simulink model "multi__micro1primarysecondarynn2"  (R2015a)
settings: Solver=ode23tb  StartTime=0.0  StopTime=2
model workspace: external: MAT-File D:\google drive\project\nn1\matla.mat (data not in the file)
undefined symbols (not defined in the file): cf, gam, gamp, k1, k2, k3, k5, Lc, lf, mp1, Mu, nq1, rc, sig, sigp, td, wn
libraries: powerlib x116, powerlib_meascontrol x32, powerlib_extras x2
(part 2 of 3)

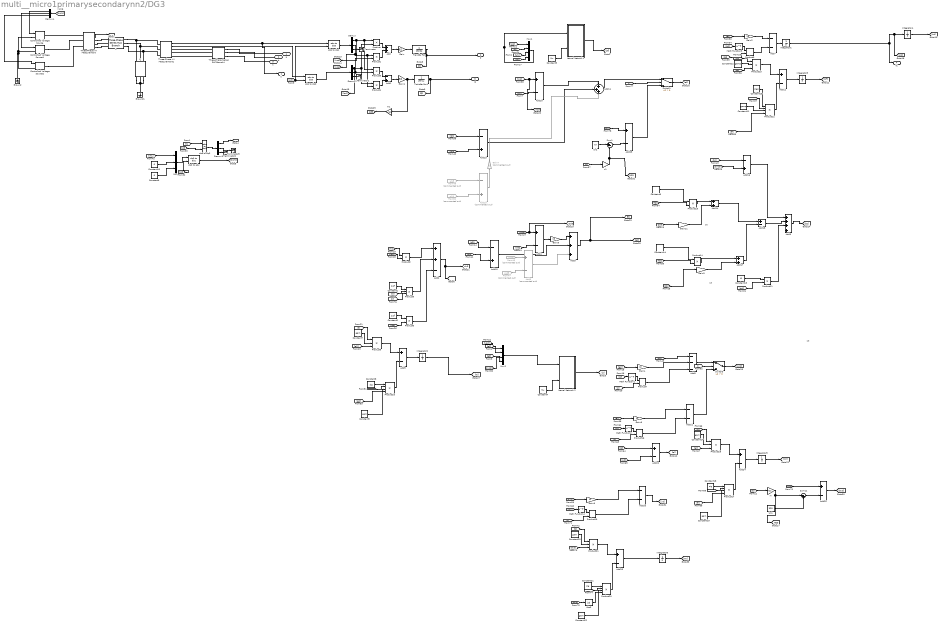
== system multi__micro1primarysecondarynn2/DG3 ==
  note: SE
  note: SE
  note: SE
  Abs3 : Abs
  Add : Sum
  Add{1,13,15..16} (4 alike) : Sum  Inputs=-+
  Add{4,9..10,12,18,22..26} (10 alike) : Sum  Inputs=+-
  Add11 : Sum  Inputs=+++
  Add14 : Sum
  Add17 : Sum
  Add19 : Sum  Commented=on  Inputs=-+
  Add2 : Sum  Inputs=++-
  Add20 : Sum  Inputs=--
  Add21 : Sum  Inputs=--
  Add3 : Sum  Inputs=+++
  Add5 : Sum  Inputs=++++
  Add6 : Sum  Commented=on  Inputs=+-
  Add7 : Sum  Inputs=--
  Add8 : Sum  Inputs=---
  C : powerlib/Elements/Three-Phase Series RLC Branch  LConnTagsString=A|B|C  RConnTagsString=A|B|C  BranchType=C  Resistance=1  Inductance=1e-3  Capacitance=cf  Measurements=None
  Constant1 : Constant  Value=1/cf
  Constant10 : Constant  Value=0
  Constant11 : Constant  Value=gamp
  Constant12 : Constant  Value=gamp
  Constant13 : Constant  Value=sigp
  Constant14 : Constant  Value=-31.446
  Constant15 : Constant  Value=k1
  Constant{7,9,17,19..20,22} (6 alike) : Constant  Value=gam
  Constant18 : Constant  Value=sig
  Constant2 : Constant  Value=1/cf
  Constant21 : Constant  Value=sig
  Constant3 : Constant  Value=Mu
  Constant4 : Constant  Value=Mu
  Constant5 : Constant  Value=-31.446
  Constant6 : Constant  Value=0
  Constant8 : Constant  Value=sig
  Controlled Voltage Source : powerlib/Electrical Sources/Controlled Voltage Source  Initialize=on  Source_Type=AC  Amplitude=0  Phase=0  Frequency=0  Measurements=None
  Controlled Voltage Source1 : powerlib/Electrical Sources/Controlled Voltage Source  Initialize=on  Source_Type=AC  Amplitude=0  Phase=0  Frequency=0  Measurements=None
  Controlled Voltage Source2 : powerlib/Electrical Sources/Controlled Voltage Source  Initialize=on  Source_Type=AC  Amplitude=0  Phase=0  Frequency=0  Measurements=None
  Demux{,1,3..4} (4 alike) : Demux  Outputs=3
  From46 : From  Commented=on  GotoTag=vod
  From47 : From  Commented=on  GotoTag=vod8
  From49 : From  Commented=on  GotoTag=w18  TagVisibility=global
  From52 : From  Commented=on  GotoTag=w11  TagVisibility=global
  Gain : Gain  Gain=3/2
  Gain1 : Gain  Gain=3/2
  Gain11 : Gain  Gain=31.446
  Gain2 : Gain  Gain=k3
  Gain3 : Gain  Gain=31.446
  Gain4 : Gain  Gain=k2
  Gain5 : Gain  Gain=k5
  Gain7 : Gain  Commented=on  Gain=k5
  Gain8 : Gain  Gain=k2
  Gain9 : Gain  Gain=k2
  Ground : powerlib/Elements/Ground  LConnTagsString=a
  Ground1 : powerlib/Elements/Ground  LConnTagsString=a
  Integrator1 : Integrator  UpperSaturationLimit=321  LowerSaturationLimit=314.16
  Integrator{2..3,5..6} (4 alike) : Integrator  InitialCondition=zeros(16,1)  UpperSaturationLimit=314.16  ZeroCross=off
  Integrator4 : Integrator  UpperSaturationLimit=314.16  ZeroCross=off
  L : powerlib/Elements/Three-Phase Series RLC Branch  LConnTagsString=A|B|C  RConnTagsString=A|B|C  BranchType=RL  Resistance=0.1  Inductance=lf  Capacitance=1e-6  Measurements=None
  Math Function{1..4} (4 alike) : Math  Operator=transpose  OutputSignalType=real  SaturateOnIntegerOverflow=on
  Mux : Mux  Inputs=3
  Mux1 : Mux
  Mux2 : Mux
  Neural Network 1 : MATLAB Function  TreatAsAtomicUnit=on
  Neural Network 2 : MATLAB Function  TreatAsAtomicUnit=on
  Product{,1,3..4} (4 alike) : Product  RndMeth=Zero
  Product{10,12,17,20} (4 alike) : Product  Inputs=4
  Product{2,6,11,14..15} (5 alike) : Product
  Product{5,8,13,18,21} (5 alike) : Product  Inputs=3
  Product{7,9,16,19} (4 alike) : Product  Multiplication=Matrix(*)
  Sum1 : Sum  Inputs=|+-
  Sum11 : Sum  Inputs=|-+
  Switch1 : Switch  Criteria=u2 > Threshold
  Switch3 : Switch  Criteria=u2 > Threshold
  Terminator{,1..3} (4 alike) : Terminator
  Three-Phase Series RLC Branch4 : powerlib/Elements/Three-Phase Series RLC Branch  LConnTagsString=A|B|C  RConnTagsString=A|B|C  BranchType=RL  Resistance=rc  Inductance=Lc  Capacitance=1e-6  Measurements=None
  Three-Phase V-I Measurement : powerlib/Measurements/Three-Phase V-I Measurement  VoltageMeasurement=phase-to-ground  SetLabelV=off  LabelV=Vabc  Vpu=off  VpuLL=off  CurrentMeasurement=yes  SetLabelI=off  LabelI=Iabc  Ipu=off  Pbase=100e6  Vbase=500e3  OutputType=Complex  PhasorSimulation=off  PSBequivalent=0
  Three-Phase V-I Measurement1 : powerlib/Measurements/Three-Phase V-I Measurement  VoltageMeasurement=phase-to-ground  SetLabelV=off  LabelV=Vabc  Vpu=off  VpuLL=off  CurrentMeasurement=yes  SetLabelI=off  LabelI=Iabc  Ipu=off  Pbase=100e6  Vbase=500e3  OutputType=Complex  PhasorSimulation=off  PSBequivalent=0
  Transfer Fcn : TransferFcn  Denominator=[td 1]
  Transfer Fcn1 : TransferFcn  Denominator=[td 1]
  Un1 : Constant  Value=325
  Un2 : Constant  Value=wn
  abc to dq0 : powerlib_meascontrol/Transformations/abc to dq0  Alignment=90 degrees behind phase A axis
  abc to dq1 : powerlib_meascontrol/Transformations/abc to dq0  Alignment=90 degrees behind phase A axis
  abc to dq3 : powerlib_meascontrol/Transformations/abc to dq0  Alignment=90 degrees behind phase A axis
  dq0 to abc : powerlib_meascontrol/Transformations/dq0 to abc  Alignment=90 degrees behind phase A axis
  m : Gain  Gain=nq1
  m1 : Gain  Gain=nq1
  n1 : Gain  Gain=mp1
  a : PMIOPort  Tag=PMCPort  Port=1  Side=Right
  b : PMIOPort  Tag=PMCPort  Port=2  Side=Right
  c : PMIOPort  Tag=PMCPort  Port=3  Side=Right
  U : Outport
  P : Outport  Port=2
  Q : Outport  Port=3
  f1 : Outport  Port=4
  tag scope: E3=global, MP3=global, NQ3=global, Q33=global, dv3=global, vod3=global, w13=global
  wires:
  [PWM] -> Demux4/1
  Three-Phase V-I Measurement1/1 -> U/1, abc to dq1/1
  Demux/1 -> [vod], Product/1, Product3/1
  Demux1/1 -> [iod], Product/2, Product4/1
  Demux/2 -> [voq], Product1/1, Product4/2
  Demux1/2 -> Product1/2, Product3/2
  Product/1 -> Add/1
  Product1/1 -> Add/2
  Product3/1 -> Add1/1
  Product4/1 -> Add1/2
  [wt] -> abc to dq1/2, abc to dq0/2
  Demux4/1 -> Controlled Voltage Source/1
  Demux4/2 -> Controlled Voltage Source1/1
  Demux4/3 -> Controlled Voltage Source2/1
  Three-Phase V-I Measurement/2 -> [IL]
  Add/1 -> Gain/1
  Gain/1 -> Transfer Fcn/1
  Add1/1 -> Gain1/1
  Gain1/1 -> m1/1, Transfer Fcn1/1
  abc to dq1/1 -> Demux/1
  abc to dq0/1 -> Demux1/1
  Demux/3 -> Terminator/1
  Demux1/3 -> Terminator1/1
  [vod] -> [vod3], Add4/1
  Gain4/1 -> Add8/2
  [e2] -> Gain4/1
  [S] -> Product7/2
  [W] -> Math Function1/1
  Math Function1/1 -> Product7/1
  Product7/1 -> Add8/3
  [S] -> Product8/1
  Constant7/1 -> Product8/2
  [e2] -> Product8/3
  Product8/1 -> Add9/1
  Constant8/1 -> Product10/1
  [W] -> Product10/2
  Product10/1 -> Add9/2
  Constant9/1 -> Product10/3
  Add9/1 -> Integrator2/1
  [vod2] -> Add4/2
  [IL] -> abc to dq3/1
  Demux3/1 -> [Id]
  Demux3/2 -> Terminator3/1
  [wt] -> abc to dq3/2
  Mux/1 -> dq0 to abc/1
  [wt] -> dq0 to abc/2
  abc to dq3/1 -> Demux3/1
  dq0 to abc/1 -> [PWM]
  Demux3/3 -> Terminator2/1
  [vn1] -> Mux/1
  Constant10/1 -> Mux/2
  Constant6/1 -> Mux/3
  Transfer Fcn/1 -> P/1, [P]
  Transfer Fcn1/1 -> Q/1, [Q]
  [w1] -> Mux1/1
  [ef] -> Mux1/2
  [w1] -> Mux1/3
  [MP2] -> Mux1/4
  [w1] -> [w13], Add10/1
  [w12] -> Add10/2
  [Sf] -> Product13/1
  Constant12/1 -> Product13/2
  [ef] -> Product13/3
  Product13/1 -> Add12/1
  Constant13/1 -> Product12/1
  [Wf] -> Product12/2
  Product12/1 -> Add12/2
  Constant11/1 -> Product12/3
  Add12/1 -> Integrator3/1
  Integrator3/1 -> [Wf]
  Three-Phase V-I Measurement1/2 -> abc to dq0/1
  Add10/1 -> Add11/1
  [MP2] -> Add13/1
  [MP3] -> Add13/2
  Add13/1 -> Add11/2
  [NQ2] -> Add15/1
  [NQ3] -> Add15/2
  Add15/1 -> Add3/2
  [e1] -> Add8/1
  Add4/1 -> Gain5/1
  Gain5/1 -> Add3/1
  [vod] -> Mux2/1
  [e1] -> Mux2/2
  [dvodi] -> Mux2/3
  [e2] -> Mux2/4
  Constant5/1 -> Product15/1
  [NQ3] -> Product15/2
  Product15/1 -> Add14/1
  [Q33] -> Gain11/1
  Constant14/1 -> Product14/1
  [NQ2] -> Product14/2
  Product14/1 -> Add17/1
  [Q22] -> Gain3/1
  Add17/1 -> Add18/2
  Add14/1 -> Add18/1
  Gain3/1 -> Add17/2
  Gain11/1 -> Add14/2
  Add18/1 -> Add5/2
  Constant15/1 -> Product11/1
  [e1] -> Product11/2
  Product11/1 -> Add5/3
  [dv2] -> Add16/1
  Add16/1 -> Add5/1
  [dvodi] -> Add16/2
  From46/1 -> Add6/1
  From47/1 -> Add6/2
  Add6/1 -> Add3/3
  m1/1 -> [Q33]
  From49/1 -> Add19/1
  From52/1 -> Add19/2
  Add19/1 -> Gain7/1
  Gain7/1 -> Add11/3
  Neural Network 1/1(Sz1) -> [Sf]
  [e2] -> Product10/4
  [ef] -> Gain2/1
  [Sf] -> Product9/2
  [Wf] -> Math Function3/1
  Math Function3/1 -> Product9/1
  Gain2/1 -> Add7/1
  Product9/1 -> Add7/2
  Add7/1 -> Integrator1/1
  [ef] -> Product12/4
  Neural Network 2/1(Sz1) -> [S]
  Constant4/1 -> Neural Network 2/2(mu)
  Mux2/1 -> Neural Network 2/1(X)
  Constant3/1 -> Neural Network 1/2(mu)
  Mux1/1 -> Neural Network 1/1(X)
  Add3/1 -> [E3], [e1]
  Add5/1 -> [e2]
  Integrator4/1 -> [wt]
  [ti] -> Switch3/2
  Add8/1 -> Switch3/1
  Switch3/1 -> [vn1]
  [el] -> Gain8/1
  [S] -> Product16/2
  [Wl] -> Math Function2/1
  Math Function2/1 -> Product16/1
  Product16/1 -> Add21/2
  Gain8/1 -> Add21/1
  Add21/1 -> Switch3/3
  [Id] -> Add22/1
  [vd] -> Add22/2
  Add22/1 -> [el]
  [S] -> Product18/1
  Constant17/1 -> Product18/2
  [el] -> Product18/3
  Product18/1 -> Add24/1
  Constant18/1 -> Product17/1
  [Wl] -> Product17/2
  Product17/1 -> Add24/2
  Constant19/1 -> Product17/3
  Add24/1 -> Integrator5/1
  Integrator5/1 -> [Wl]
  [el] -> Product17/4
  [vod] -> Add25/1
  Add25/1 -> [evd]
  Sum11/1 -> Add25/2
  [Q] -> m/1
  Un1/1 -> Sum11/2
  m/1 -> [NQ3], Sum11/1
  [evd] -> Gain9/1
  [S] -> Product19/2
  [Wv] -> Math Function4/1
  Math Function4/1 -> Product19/1
  Product19/1 -> Add20/2
  Gain9/1 -> Add20/1
  Add20/1 -> [vd]
  [S] -> Product21/1
  Constant20/1 -> Product21/2
  [evd] -> Product21/3
  Product21/1 -> Add26/1
  Constant21/1 -> Product20/1
  [Wl] -> Product20/2
  Product20/1 -> Add26/2
  Constant22/1 -> Product20/3
  Abs3/1 -> Product20/4
  [evd] -> Abs3/1
  Add26/1 -> Integrator6/1
  Integrator6/1 -> [Wv]
  Integrator2/1 -> [W]
  [w1] -> Product2/1
  [voq] -> Product2/2
  Product2/1 -> Add2/1
  Constant1/1 -> Product5/1
  [Id] -> Product5/2
  Product5/1 -> Add2/2
  Constant2/1 -> Product6/1
  [iod] -> Product6/2
  Product6/1 -> Add2/3
  Add2/1 -> [dvodi], [dv3]
  [rr] -> Product5/3
  Integrator1/1 -> [w1], Integrator4/1, f1/1
  [P] -> n1/1
  Un2/1 -> Sum1/1  "f"
  n1/1 -> [MP3], Sum1/2
  Sum1/1 -> Add23/2
  [w1] -> Add23/1
  Add11/1 -> Switch1/1
  [ti] -> Switch1/2
  Switch1/1 -> [ef]
  Add23/1 -> Switch1/3
  connections:
  C/RConn1 -- Ground1/LConn1 -- C/RConn3 -- C/RConn2
  L/RConn2 -- Three-Phase V-I Measurement1/LConn2 -- C/LConn2
  L/RConn1 -- Three-Phase V-I Measurement1/LConn1 -- C/LConn1
  L/RConn3 -- Three-Phase V-I Measurement1/LConn3 -- C/LConn3
  Controlled Voltage Source/LConn1 -- Controlled Voltage Source1/LConn1 -- Ground/LConn1 -- Controlled Voltage Source2/LConn1
  Three-Phase V-I Measurement/LConn1 -- Controlled Voltage Source/RConn1
  Controlled Voltage Source1/RConn1 -- Three-Phase V-I Measurement/LConn2
  Controlled Voltage Source2/RConn1 -- Three-Phase V-I Measurement/LConn3
  Three-Phase V-I Measurement/RConn1 -- L/LConn1
  Three-Phase V-I Measurement/RConn2 -- L/LConn2
  Three-Phase V-I Measurement/RConn3 -- L/LConn3
  Three-Phase Series RLC Branch4/RConn1 -- Three-Phase V-I Measurement1/RConn1
  Three-Phase Series RLC Branch4/RConn2 -- Three-Phase V-I Measurement1/RConn2
  Three-Phase Series RLC Branch4/RConn3 -- Three-Phase V-I Measurement1/RConn3
  Three-Phase Series RLC Branch4/LConn3 -- c/RConn1
  Three-Phase Series RLC Branch4/LConn2 -- b/RConn1
  Three-Phase Series RLC Branch4/LConn1 -- a/RConn1

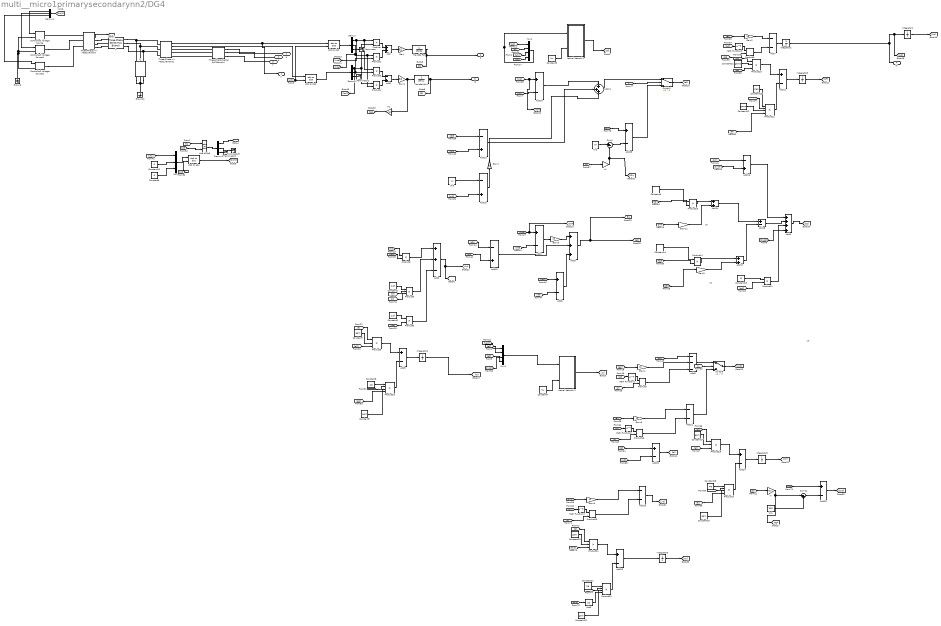
== system multi__micro1primarysecondarynn2/DG4 ==
  note: SE
  note: SE
  note: SE
  Abs3 : Abs
  Add : Sum
  Add{1,13,15..16,19} (5 alike) : Sum  Inputs=-+
  Add{4,6,9..10,12,18,22..26} (11 alike) : Sum  Inputs=+-
  Add11 : Sum  Inputs=+++
  Add14 : Sum
  Add17 : Sum
  Add2 : Sum  Inputs=++-
  Add20 : Sum  Inputs=--
  Add21 : Sum  Inputs=--
  Add3 : Sum  Inputs=+++
  Add5 : Sum  Inputs=++++
  Add7 : Sum  Inputs=--
  Add8 : Sum  Inputs=---
  C : powerlib/Elements/Three-Phase Series RLC Branch  LConnTagsString=A|B|C  RConnTagsString=A|B|C  BranchType=C  Resistance=1  Inductance=1e-3  Capacitance=cf  Measurements=None
  Constant1 : Constant  Value=1/cf
  Constant10 : Constant  Value=0
  Constant11 : Constant  Value=gamp
  Constant12 : Constant  Value=gamp
  Constant13 : Constant  Value=sigp
  Constant14 : Constant  Value=-31.446
  Constant15 : Constant  Value=k1
  Constant{7,9,17,19..20,22} (6 alike) : Constant  Value=gam
  Constant18 : Constant  Value=sig
  Constant2 : Constant  Value=1/cf
  Constant21 : Constant  Value=sig
  Constant3 : Constant  Value=Mu
  Constant4 : Constant  Value=Mu
  Constant5 : Constant  Value=-31.446
  Constant6 : Constant  Value=0
  Constant8 : Constant  Value=sig
  Controlled Voltage Source : powerlib/Electrical Sources/Controlled Voltage Source  Initialize=on  Source_Type=AC  Amplitude=0  Phase=0  Frequency=0  Measurements=None
  Controlled Voltage Source1 : powerlib/Electrical Sources/Controlled Voltage Source  Initialize=on  Source_Type=AC  Amplitude=0  Phase=0  Frequency=0  Measurements=None
  Controlled Voltage Source2 : powerlib/Electrical Sources/Controlled Voltage Source  Initialize=on  Source_Type=AC  Amplitude=0  Phase=0  Frequency=0  Measurements=None
  Demux{,1,3..4} (4 alike) : Demux  Outputs=3
  Gain : Gain  Gain=3/2
  Gain1 : Gain  Gain=3/2
  Gain11 : Gain  Gain=31.446
  Gain2 : Gain  Gain=k3
  Gain3 : Gain  Gain=31.446
  Gain4 : Gain  Gain=k2
  Gain5 : Gain  Gain=k5
  Gain7 : Gain  Gain=k5
  Gain8 : Gain  Gain=k2
  Gain9 : Gain  Gain=k2
  Ground : powerlib/Elements/Ground  LConnTagsString=a
  Ground1 : powerlib/Elements/Ground  LConnTagsString=a
  Integrator1 : Integrator  UpperSaturationLimit=321  LowerSaturationLimit=314.16
  Integrator{2..3,5..6} (4 alike) : Integrator  InitialCondition=zeros(16,1)  UpperSaturationLimit=314.16  ZeroCross=off
  Integrator4 : Integrator  UpperSaturationLimit=314.16  ZeroCross=off
  L : powerlib/Elements/Three-Phase Series RLC Branch  LConnTagsString=A|B|C  RConnTagsString=A|B|C  BranchType=RL  Resistance=0.1  Inductance=lf  Capacitance=1e-6  Measurements=None
  Math Function{1..4} (4 alike) : Math  Operator=transpose  OutputSignalType=real  SaturateOnIntegerOverflow=on
  Mux : Mux  Inputs=3
  Mux1 : Mux
  Mux2 : Mux
  Neural Network 1 : MATLAB Function  TreatAsAtomicUnit=on
  Neural Network 2 : MATLAB Function  TreatAsAtomicUnit=on
  Product{,1,3..4} (4 alike) : Product  RndMeth=Zero
  Product{10,12,17,20} (4 alike) : Product  Inputs=4
  Product{2,6,11,14..15} (5 alike) : Product
  Product{5,8,13,18,21} (5 alike) : Product  Inputs=3
  Product{7,9,16,19} (4 alike) : Product  Multiplication=Matrix(*)
  Sum1 : Sum  Inputs=|+-
  Sum11 : Sum  Inputs=|-+
  Switch1 : Switch  Criteria=u2 > Threshold
  Switch3 : Switch  Criteria=u2 > Threshold
  Terminator{,1..3} (4 alike) : Terminator
  Three-Phase Series RLC Branch4 : powerlib/Elements/Three-Phase Series RLC Branch  LConnTagsString=A|B|C  RConnTagsString=A|B|C  BranchType=RL  Resistance=rc  Inductance=Lc  Capacitance=1e-6  Measurements=None
  Three-Phase V-I Measurement : powerlib/Measurements/Three-Phase V-I Measurement  VoltageMeasurement=phase-to-ground  SetLabelV=off  LabelV=Vabc  Vpu=off  VpuLL=off  CurrentMeasurement=yes  SetLabelI=off  LabelI=Iabc  Ipu=off  Pbase=100e6  Vbase=500e3  OutputType=Complex  PhasorSimulation=off  PSBequivalent=0
  Three-Phase V-I Measurement1 : powerlib/Measurements/Three-Phase V-I Measurement  VoltageMeasurement=phase-to-ground  SetLabelV=off  LabelV=Vabc  Vpu=off  VpuLL=off  CurrentMeasurement=yes  SetLabelI=off  LabelI=Iabc  Ipu=off  Pbase=100e6  Vbase=500e3  OutputType=Complex  PhasorSimulation=off  PSBequivalent=0
  Transfer Fcn : TransferFcn  Denominator=[td 1]
  Transfer Fcn1 : TransferFcn  Denominator=[td 1]
  Un1 : Constant  Value=325
  Un2 : Constant  Value=wn
  Un3 : Constant  Value=wn
  abc to dq0 : powerlib_meascontrol/Transformations/abc to dq0  Alignment=90 degrees behind phase A axis
  abc to dq1 : powerlib_meascontrol/Transformations/abc to dq0  Alignment=90 degrees behind phase A axis
  abc to dq3 : powerlib_meascontrol/Transformations/abc to dq0  Alignment=90 degrees behind phase A axis
  dq0 to abc : powerlib_meascontrol/Transformations/dq0 to abc  Alignment=90 degrees behind phase A axis
  m : Gain  Gain=nq1
  m1 : Gain  Gain=nq1
  n1 : Gain  Gain=mp1
  a : PMIOPort  Tag=PMCPort  Port=1  Side=Right
  b : PMIOPort  Tag=PMCPort  Port=2  Side=Right
  c : PMIOPort  Tag=PMCPort  Port=3  Side=Right
  U : Outport
  P : Outport  Port=2
  Q : Outport  Port=3
  f1 : Outport  Port=4
  tag scope: E4=global, MP4=global, NQ4=global, Q44=global, dv4=global, vod4=global, w14=global
  wires:
  [PWM] -> Demux4/1
  Three-Phase V-I Measurement1/1 -> U/1, abc to dq1/1
  Demux/1 -> [vod], Product/1, Product3/1
  Demux1/1 -> [iod], Product/2, Product4/1
  Demux/2 -> [voq], Product1/1, Product4/2
  Demux1/2 -> Product1/2, Product3/2
  Product/1 -> Add/1
  Product1/1 -> Add/2
  Product3/1 -> Add1/1
  Product4/1 -> Add1/2
  [wt] -> abc to dq1/2, abc to dq0/2
  Demux4/1 -> Controlled Voltage Source/1
  Demux4/2 -> Controlled Voltage Source1/1
  Demux4/3 -> Controlled Voltage Source2/1
  Three-Phase V-I Measurement/2 -> [IL]
  Add/1 -> Gain/1
  Gain/1 -> Transfer Fcn/1
  Add1/1 -> Gain1/1
  Gain1/1 -> m1/1, Transfer Fcn1/1
  abc to dq1/1 -> Demux/1
  abc to dq0/1 -> Demux1/1
  Demux/3 -> Terminator/1
  Demux1/3 -> Terminator1/1
  [vod] -> [vod4], Add4/1
  Gain4/1 -> Add8/2
  [e2] -> Gain4/1
  [S] -> Product7/2
  [W] -> Math Function1/1
  Math Function1/1 -> Product7/1
  Product7/1 -> Add8/3
  [S] -> Product8/1
  Constant7/1 -> Product8/2
  [e2] -> Product8/3
  Product8/1 -> Add9/1
  Constant8/1 -> Product10/1
  [W] -> Product10/2
  Product10/1 -> Add9/2
  Constant9/1 -> Product10/3
  Add9/1 -> Integrator2/1
  [vod3] -> Add4/2
  [IL] -> abc to dq3/1
  Demux3/1 -> [Id]
  Demux3/2 -> Terminator3/1
  [wt] -> abc to dq3/2
  Mux/1 -> dq0 to abc/1
  [wt] -> dq0 to abc/2
  abc to dq3/1 -> Demux3/1
  dq0 to abc/1 -> [PWM]
  Demux3/3 -> Terminator2/1
  [vn1] -> Mux/1
  Constant10/1 -> Mux/2
  Constant6/1 -> Mux/3
  Transfer Fcn/1 -> P/1, [P]
  Transfer Fcn1/1 -> Q/1, [Q]
  [w1] -> Mux1/1
  [ef] -> Mux1/2
  [w1] -> Mux1/3
  [MP2] -> Mux1/4
  [w1] -> [w14], Add10/1
  [w13] -> Add10/2
  [Sf] -> Product13/1
  Constant12/1 -> Product13/2
  [ef] -> Product13/3
  Product13/1 -> Add12/1
  Constant13/1 -> Product12/1
  [Wf] -> Product12/2
  Product12/1 -> Add12/2
  Constant11/1 -> Product12/3
  Add12/1 -> Integrator3/1
  Integrator3/1 -> [Wf]
  Three-Phase V-I Measurement1/2 -> abc to dq0/1
  Add10/1 -> Add11/1
  [MP3] -> Add13/1
  [MP4] -> Add13/2
  Add13/1 -> Add11/2
  [NQ2] -> Add15/1
  [NQ3] -> Add15/2
  Add15/1 -> Add3/2
  [e1] -> Add8/1
  Add4/1 -> Gain5/1
  Gain5/1 -> Add3/1
  [vod] -> Mux2/1
  [e1] -> Mux2/2
  [dvodi] -> Mux2/3
  [e2] -> Mux2/4
  Constant5/1 -> Product15/1
  [NQ4] -> Product15/2
  Product15/1 -> Add14/1
  [Q44] -> Gain11/1
  Constant14/1 -> Product14/1
  [NQ3] -> Product14/2
  Product14/1 -> Add17/1
  [Q33] -> Gain3/1
  Add17/1 -> Add18/2
  Add14/1 -> Add18/1
  Gain3/1 -> Add17/2
  Gain11/1 -> Add14/2
  Add18/1 -> Add5/2
  Constant15/1 -> Product11/1
  [e1] -> Product11/2
  Product11/1 -> Add5/3
  [dv3] -> Add16/1
  Add16/1 -> Add5/1
  [dvodi] -> Add16/2
  [vod] -> Add6/1
  [vref] -> Add6/2
  Add6/1 -> Add3/3
  m1/1 -> [Q44]
  Un3/1 -> Add19/1
  [w1] -> Add19/2
  Add19/1 -> Gain7/1
  Gain7/1 -> Add11/3
  Neural Network 1/1(Sz1) -> [Sf]
  [e2] -> Product10/4
  [ef] -> Gain2/1
  [Sf] -> Product9/2
  [Wf] -> Math Function3/1
  Math Function3/1 -> Product9/1
  Gain2/1 -> Add7/1
  Product9/1 -> Add7/2
  Add7/1 -> Integrator1/1
  [ef] -> Product12/4
  Neural Network 2/1(Sz1) -> [S]
  Constant4/1 -> Neural Network 2/2(mu)
  Mux2/1 -> Neural Network 2/1(X)
  Constant3/1 -> Neural Network 1/2(mu)
  Mux1/1 -> Neural Network 1/1(X)
  Add3/1 -> [E4], [e1]
  Add5/1 -> [e2]
  Integrator4/1 -> [wt]
  [ti] -> Switch3/2
  Add8/1 -> Switch3/1
  Switch3/1 -> [vn1]
  [el] -> Gain8/1
  [S] -> Product16/2
  [Wl] -> Math Function2/1
  Math Function2/1 -> Product16/1
  Product16/1 -> Add21/2
  Gain8/1 -> Add21/1
  Add21/1 -> Switch3/3
  [Id] -> Add22/1
  [vd] -> Add22/2
  Add22/1 -> [el]
  [S] -> Product18/1
  Constant17/1 -> Product18/2
  [el] -> Product18/3
  Product18/1 -> Add24/1
  Constant18/1 -> Product17/1
  [Wl] -> Product17/2
  Product17/1 -> Add24/2
  Constant19/1 -> Product17/3
  Add24/1 -> Integrator5/1
  Integrator5/1 -> [Wl]
  [el] -> Product17/4
  [vod] -> Add25/1
  Add25/1 -> [evd]
  Sum11/1 -> Add25/2
  [Q] -> m/1
  Un1/1 -> Sum11/2
  m/1 -> [NQ4], Sum11/1
  [evd] -> Gain9/1
  [S] -> Product19/2
  [Wv] -> Math Function4/1
  Math Function4/1 -> Product19/1
  Product19/1 -> Add20/2
  Gain9/1 -> Add20/1
  Add20/1 -> [vd]
  [S] -> Product21/1
  Constant20/1 -> Product21/2
  [evd] -> Product21/3
  Product21/1 -> Add26/1
  Constant21/1 -> Product20/1
  [Wl] -> Product20/2
  Product20/1 -> Add26/2
  Constant22/1 -> Product20/3
  Abs3/1 -> Product20/4
  [evd] -> Abs3/1
  Add26/1 -> Integrator6/1
  Integrator6/1 -> [Wv]
  Integrator2/1 -> [W]
  [w1] -> Product2/1
  [voq] -> Product2/2
  Product2/1 -> Add2/1
  Constant1/1 -> Product5/1
  [Id] -> Product5/2
  Product5/1 -> Add2/2
  Constant2/1 -> Product6/1
  [iod] -> Product6/2
  Product6/1 -> Add2/3
  Add2/1 -> [dvodi], [dv4]
  [rr] -> Product5/3
  Integrator1/1 -> [w1], Integrator4/1, f1/1
  [P] -> n1/1
  Un2/1 -> Sum1/1  "f"
  n1/1 -> [MP4], Sum1/2
  Sum1/1 -> Add23/2
  [w1] -> Add23/1
  Add11/1 -> Switch1/1
  [ti] -> Switch1/2
  Switch1/1 -> [ef]
  Add23/1 -> Switch1/3
  [dvodi] -> Add5/4
  connections:
  C/RConn1 -- Ground1/LConn1 -- C/RConn3 -- C/RConn2
  L/RConn2 -- Three-Phase V-I Measurement1/LConn2 -- C/LConn2
  L/RConn1 -- Three-Phase V-I Measurement1/LConn1 -- C/LConn1
  L/RConn3 -- Three-Phase V-I Measurement1/LConn3 -- C/LConn3
  Controlled Voltage Source/LConn1 -- Controlled Voltage Source1/LConn1 -- Ground/LConn1 -- Controlled Voltage Source2/LConn1
  Three-Phase V-I Measurement/LConn1 -- Controlled Voltage Source/RConn1
  Controlled Voltage Source1/RConn1 -- Three-Phase V-I Measurement/LConn2
  Controlled Voltage Source2/RConn1 -- Three-Phase V-I Measurement/LConn3
  Three-Phase V-I Measurement/RConn1 -- L/LConn1
  Three-Phase V-I Measurement/RConn2 -- L/LConn2
  Three-Phase V-I Measurement/RConn3 -- L/LConn3
  Three-Phase Series RLC Branch4/RConn1 -- Three-Phase V-I Measurement1/RConn1
  Three-Phase Series RLC Branch4/RConn2 -- Three-Phase V-I Measurement1/RConn2
  Three-Phase Series RLC Branch4/RConn3 -- Three-Phase V-I Measurement1/RConn3
  Three-Phase Series RLC Branch4/LConn3 -- c/RConn1
  Three-Phase Series RLC Branch4/LConn2 -- b/RConn1
  Three-Phase Series RLC Branch4/LConn1 -- a/RConn1

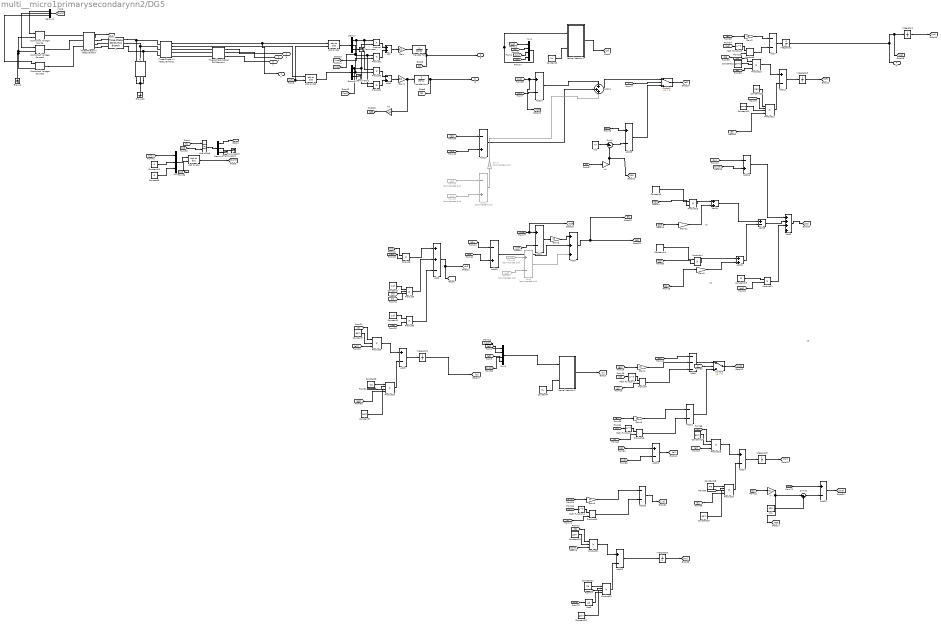
== system multi__micro1primarysecondarynn2/DG5 ==
  note: SE
  note: SE
  note: SE
  Abs3 : Abs
  Add : Sum
  Add{1,13,15..16} (4 alike) : Sum  Inputs=-+
  Add{4,9..10,12,18,22..26} (10 alike) : Sum  Inputs=+-
  Add11 : Sum  Inputs=+++
  Add14 : Sum
  Add17 : Sum
  Add19 : Sum  Commented=on  Inputs=-+
  Add2 : Sum  Inputs=++-
  Add20 : Sum  Inputs=--
  Add21 : Sum  Inputs=--
  Add3 : Sum  Inputs=+++
  Add5 : Sum  Inputs=++++
  Add6 : Sum  Commented=on  Inputs=+-
  Add7 : Sum  Inputs=--
  Add8 : Sum  Inputs=---
  C : powerlib/Elements/Three-Phase Series RLC Branch  LConnTagsString=A|B|C  RConnTagsString=A|B|C  BranchType=C  Resistance=1  Inductance=1e-3  Capacitance=cf  Measurements=None
  Constant1 : Constant  Value=1/cf
  Constant10 : Constant  Value=0
  Constant11 : Constant  Value=gamp
  Constant12 : Constant  Value=gamp
  Constant13 : Constant  Value=sigp
  Constant14 : Constant  Value=-31.446
  Constant15 : Constant  Value=k1
  Constant{7,9,17,19..20,22} (6 alike) : Constant  Value=gam
  Constant18 : Constant  Value=sig
  Constant2 : Constant  Value=1/cf
  Constant21 : Constant  Value=sig
  Constant3 : Constant  Value=Mu
  Constant4 : Constant  Value=Mu
  Constant5 : Constant  Value=-31.446
  Constant6 : Constant  Value=0
  Constant8 : Constant  Value=sig
  Controlled Voltage Source : powerlib/Electrical Sources/Controlled Voltage Source  Initialize=on  Source_Type=AC  Amplitude=0  Phase=0  Frequency=0  Measurements=None
  Controlled Voltage Source1 : powerlib/Electrical Sources/Controlled Voltage Source  Initialize=on  Source_Type=AC  Amplitude=0  Phase=0  Frequency=0  Measurements=None
  Controlled Voltage Source2 : powerlib/Electrical Sources/Controlled Voltage Source  Initialize=on  Source_Type=AC  Amplitude=0  Phase=0  Frequency=0  Measurements=None
  Demux{,1,3..4} (4 alike) : Demux  Outputs=3
  From46 : From  Commented=on  GotoTag=vod
  From47 : From  Commented=on  GotoTag=vod8
  From49 : From  Commented=on  GotoTag=w18  TagVisibility=global
  From52 : From  Commented=on  GotoTag=w11  TagVisibility=global
  Gain : Gain  Gain=3/2
  Gain1 : Gain  Gain=3/2
  Gain11 : Gain  Gain=31.446
  Gain2 : Gain  Gain=k3
  Gain3 : Gain  Gain=31.446
  Gain4 : Gain  Gain=k2
  Gain5 : Gain  Gain=k5
  Gain7 : Gain  Commented=on  Gain=k5
  Gain8 : Gain  Gain=k2
  Gain9 : Gain  Gain=k2
  Ground : powerlib/Elements/Ground  LConnTagsString=a
  Ground1 : powerlib/Elements/Ground  LConnTagsString=a
  Integrator1 : Integrator  UpperSaturationLimit=321  LowerSaturationLimit=314.16
  Integrator{2..3,5..6} (4 alike) : Integrator  InitialCondition=zeros(16,1)  UpperSaturationLimit=314.16  ZeroCross=off
  Integrator4 : Integrator  UpperSaturationLimit=314.16  ZeroCross=off
  L : powerlib/Elements/Three-Phase Series RLC Branch  LConnTagsString=A|B|C  RConnTagsString=A|B|C  BranchType=RL  Resistance=0.1  Inductance=lf  Capacitance=1e-6  Measurements=None
  Math Function{1..4} (4 alike) : Math  Operator=transpose  OutputSignalType=real  SaturateOnIntegerOverflow=on
  Mux : Mux  Inputs=3
  Mux1 : Mux
  Mux2 : Mux
  Neural Network 1 : MATLAB Function  TreatAsAtomicUnit=on
  Neural Network 2 : MATLAB Function  TreatAsAtomicUnit=on
  Product{,1,3..4} (4 alike) : Product  RndMeth=Zero
  Product{10,12,17,20} (4 alike) : Product  Inputs=4
  Product{2,6,11,14..15} (5 alike) : Product
  Product{5,8,13,18,21} (5 alike) : Product  Inputs=3
  Product{7,9,16,19} (4 alike) : Product  Multiplication=Matrix(*)
  Sum1 : Sum  Inputs=|+-
  Sum11 : Sum  Inputs=|-+
  Switch1 : Switch  Criteria=u2 > Threshold
  Switch3 : Switch  Criteria=u2 > Threshold
  Terminator{,1..3} (4 alike) : Terminator
  Three-Phase Series RLC Branch4 : powerlib/Elements/Three-Phase Series RLC Branch  LConnTagsString=A|B|C  RConnTagsString=A|B|C  BranchType=RL  Resistance=rc  Inductance=Lc  Capacitance=1e-6  Measurements=None
  Three-Phase V-I Measurement : powerlib/Measurements/Three-Phase V-I Measurement  VoltageMeasurement=phase-to-ground  SetLabelV=off  LabelV=Vabc  Vpu=off  VpuLL=off  CurrentMeasurement=yes  SetLabelI=off  LabelI=Iabc  Ipu=off  Pbase=100e6  Vbase=500e3  OutputType=Complex  PhasorSimulation=off  PSBequivalent=0
  Three-Phase V-I Measurement1 : powerlib/Measurements/Three-Phase V-I Measurement  VoltageMeasurement=phase-to-ground  SetLabelV=off  LabelV=Vabc  Vpu=off  VpuLL=off  CurrentMeasurement=yes  SetLabelI=off  LabelI=Iabc  Ipu=off  Pbase=100e6  Vbase=500e3  OutputType=Complex  PhasorSimulation=off  PSBequivalent=0
  Transfer Fcn : TransferFcn  Denominator=[td 1]
  Transfer Fcn1 : TransferFcn  Denominator=[td 1]
  Un1 : Constant  Value=325
  Un2 : Constant  Value=wn
  abc to dq0 : powerlib_meascontrol/Transformations/abc to dq0  Alignment=90 degrees behind phase A axis
  abc to dq1 : powerlib_meascontrol/Transformations/abc to dq0  Alignment=90 degrees behind phase A axis
  abc to dq3 : powerlib_meascontrol/Transformations/abc to dq0  Alignment=90 degrees behind phase A axis
  dq0 to abc : powerlib_meascontrol/Transformations/dq0 to abc  Alignment=90 degrees behind phase A axis
  m : Gain  Gain=nq1
  m1 : Gain  Gain=nq1
  n1 : Gain  Gain=mp1
  a : PMIOPort  Tag=PMCPort  Port=1  Side=Right
  b : PMIOPort  Tag=PMCPort  Port=2  Side=Right
  c : PMIOPort  Tag=PMCPort  Port=3  Side=Right
  U : Outport
  P : Outport  Port=2
  Q : Outport  Port=3
  f1 : Outport  Port=4
  tag scope: E5=global, MP5=global, NQ5=global, Q55=global, dv5=global, vod5=global, w15=global
  wires:
  [PWM] -> Demux4/1
  Three-Phase V-I Measurement1/1 -> U/1, abc to dq1/1
  Demux/1 -> [vod], Product/1, Product3/1
  Demux1/1 -> [iod], Product/2, Product4/1
  Demux/2 -> [voq], Product1/1, Product4/2
  Demux1/2 -> Product1/2, Product3/2
  Product/1 -> Add/1
  Product1/1 -> Add/2
  Product3/1 -> Add1/1
  Product4/1 -> Add1/2
  [wt] -> abc to dq1/2, abc to dq0/2
  Demux4/1 -> Controlled Voltage Source/1
  Demux4/2 -> Controlled Voltage Source1/1
  Demux4/3 -> Controlled Voltage Source2/1
  Three-Phase V-I Measurement/2 -> [IL]
  Add/1 -> Gain/1
  Gain/1 -> Transfer Fcn/1
  Add1/1 -> Gain1/1
  Gain1/1 -> m1/1, Transfer Fcn1/1
  abc to dq1/1 -> Demux/1
  abc to dq0/1 -> Demux1/1
  Demux/3 -> Terminator/1
  Demux1/3 -> Terminator1/1
  [vod] -> [vod5], Add4/1
  Gain4/1 -> Add8/2
  [e2] -> Gain4/1
  [S] -> Product7/2
  [W] -> Math Function1/1
  Math Function1/1 -> Product7/1
  Product7/1 -> Add8/3
  [S] -> Product8/1
  Constant7/1 -> Product8/2
  [e2] -> Product8/3
  Product8/1 -> Add9/1
  Constant8/1 -> Product10/1
  [W] -> Product10/2
  Product10/1 -> Add9/2
  Constant9/1 -> Product10/3
  Add9/1 -> Integrator2/1
  [vod4] -> Add4/2
  [IL] -> abc to dq3/1
  Demux3/1 -> [Id]
  Demux3/2 -> Terminator3/1
  [wt] -> abc to dq3/2
  Mux/1 -> dq0 to abc/1
  [wt] -> dq0 to abc/2
  abc to dq3/1 -> Demux3/1
  dq0 to abc/1 -> [PWM]
  Demux3/3 -> Terminator2/1
  [vn1] -> Mux/1
  Constant10/1 -> Mux/2
  Constant6/1 -> Mux/3
  Transfer Fcn/1 -> P/1, [P]
  Transfer Fcn1/1 -> Q/1, [Q]
  [w1] -> Mux1/1
  [ef] -> Mux1/2
  [w1] -> Mux1/3
  [MP2] -> Mux1/4
  [w1] -> [w15], Add10/1
  [w14] -> Add10/2
  [Sf] -> Product13/1
  Constant12/1 -> Product13/2
  [ef] -> Product13/3
  Product13/1 -> Add12/1
  Constant13/1 -> Product12/1
  [Wf] -> Product12/2
  Product12/1 -> Add12/2
  Constant11/1 -> Product12/3
  Add12/1 -> Integrator3/1
  Integrator3/1 -> [Wf]
  Three-Phase V-I Measurement1/2 -> abc to dq0/1
  Add10/1 -> Add11/1
  [MP4] -> Add13/1
  [MP5] -> Add13/2
  Add13/1 -> Add11/2
  [NQ4] -> Add15/1
  [NQ5] -> Add15/2
  Add15/1 -> Add3/2
  [e1] -> Add8/1
  Add4/1 -> Gain5/1
  Gain5/1 -> Add3/1
  [vod] -> Mux2/1
  [e1] -> Mux2/2
  [dvodi] -> Mux2/3
  [e2] -> Mux2/4
  Constant5/1 -> Product15/1
  [NQ5] -> Product15/2
  Product15/1 -> Add14/1
  [Q55] -> Gain11/1
  Constant14/1 -> Product14/1
  [NQ4] -> Product14/2
  Product14/1 -> Add17/1
  [Q44] -> Gain3/1
  Add17/1 -> Add18/2
  Add14/1 -> Add18/1
  Gain3/1 -> Add17/2
  Gain11/1 -> Add14/2
  Add18/1 -> Add5/2
  Constant15/1 -> Product11/1
  [e1] -> Product11/2
  Product11/1 -> Add5/3
  [dv4] -> Add16/1
  Add16/1 -> Add5/1
  [dvodi] -> Add16/2
  From46/1 -> Add6/1
  From47/1 -> Add6/2
  Add6/1 -> Add3/3
  m1/1 -> [Q55]
  From49/1 -> Add19/1
  From52/1 -> Add19/2
  Add19/1 -> Gain7/1
  Gain7/1 -> Add11/3
  Neural Network 1/1(Sz1) -> [Sf]
  [e2] -> Product10/4
  [ef] -> Gain2/1
  [Sf] -> Product9/2
  [Wf] -> Math Function3/1
  Math Function3/1 -> Product9/1
  Gain2/1 -> Add7/1
  Product9/1 -> Add7/2
  Add7/1 -> Integrator1/1
  [ef] -> Product12/4
  Neural Network 2/1(Sz1) -> [S]
  Constant4/1 -> Neural Network 2/2(mu)
  Mux2/1 -> Neural Network 2/1(X)
  Constant3/1 -> Neural Network 1/2(mu)
  Mux1/1 -> Neural Network 1/1(X)
  Add3/1 -> [E5], [e1]
  Add5/1 -> [e2]
  Integrator4/1 -> [wt]
  [ti] -> Switch3/2
  Add8/1 -> Switch3/1
  Switch3/1 -> [vn1]
  [el] -> Gain8/1
  [S] -> Product16/2
  [Wl] -> Math Function2/1
  Math Function2/1 -> Product16/1
  Product16/1 -> Add21/2
  Gain8/1 -> Add21/1
  Add21/1 -> Switch3/3
  [Id] -> Add22/1
  [vd] -> Add22/2
  Add22/1 -> [el]
  [S] -> Product18/1
  Constant17/1 -> Product18/2
  [el] -> Product18/3
  Product18/1 -> Add24/1
  Constant18/1 -> Product17/1
  [Wl] -> Product17/2
  Product17/1 -> Add24/2
  Constant19/1 -> Product17/3
  Add24/1 -> Integrator5/1
  Integrator5/1 -> [Wl]
  [el] -> Product17/4
  [vod] -> Add25/1
  Add25/1 -> [evd]
  Sum11/1 -> Add25/2
  [Q] -> m/1
  Un1/1 -> Sum11/2
  m/1 -> [NQ5], Sum11/1
  [evd] -> Gain9/1
  [S] -> Product19/2
  [Wv] -> Math Function4/1
  Math Function4/1 -> Product19/1
  Product19/1 -> Add20/2
  Gain9/1 -> Add20/1
  Add20/1 -> [vd]
  [S] -> Product21/1
  Constant20/1 -> Product21/2
  [evd] -> Product21/3
  Product21/1 -> Add26/1
  Constant21/1 -> Product20/1
  [Wl] -> Product20/2
  Product20/1 -> Add26/2
  Constant22/1 -> Product20/3
  Abs3/1 -> Product20/4
  [evd] -> Abs3/1
  Add26/1 -> Integrator6/1
  Integrator6/1 -> [Wv]
  Integrator2/1 -> [W]
  [w1] -> Product2/1
  [voq] -> Product2/2
  Product2/1 -> Add2/1
  Constant1/1 -> Product5/1
  [Id] -> Product5/2
  Product5/1 -> Add2/2
  Constant2/1 -> Product6/1
  [iod] -> Product6/2
  Product6/1 -> Add2/3
  Add2/1 -> [dvodi], [dv5]
  [rr] -> Product5/3
  Integrator1/1 -> [w1], Integrator4/1, f1/1
  [P] -> n1/1
  Un2/1 -> Sum1/1  "f"
  n1/1 -> [MP5], Sum1/2
  Sum1/1 -> Add23/2
  [w1] -> Add23/1
  Add11/1 -> Switch1/1
  [ti] -> Switch1/2
  Switch1/1 -> [ef]
  Add23/1 -> Switch1/3
  connections:
  C/RConn1 -- Ground1/LConn1 -- C/RConn3 -- C/RConn2
  L/RConn2 -- Three-Phase V-I Measurement1/LConn2 -- C/LConn2
  L/RConn1 -- Three-Phase V-I Measurement1/LConn1 -- C/LConn1
  L/RConn3 -- Three-Phase V-I Measurement1/LConn3 -- C/LConn3
  Controlled Voltage Source/LConn1 -- Controlled Voltage Source1/LConn1 -- Ground/LConn1 -- Controlled Voltage Source2/LConn1
  Three-Phase V-I Measurement/LConn1 -- Controlled Voltage Source/RConn1
  Controlled Voltage Source1/RConn1 -- Three-Phase V-I Measurement/LConn2
  Controlled Voltage Source2/RConn1 -- Three-Phase V-I Measurement/LConn3
  Three-Phase V-I Measurement/RConn1 -- L/LConn1
  Three-Phase V-I Measurement/RConn2 -- L/LConn2
  Three-Phase V-I Measurement/RConn3 -- L/LConn3
  Three-Phase Series RLC Branch4/RConn1 -- Three-Phase V-I Measurement1/RConn1
  Three-Phase Series RLC Branch4/RConn2 -- Three-Phase V-I Measurement1/RConn2
  Three-Phase Series RLC Branch4/RConn3 -- Three-Phase V-I Measurement1/RConn3
  Three-Phase Series RLC Branch4/LConn3 -- c/RConn1
  Three-Phase Series RLC Branch4/LConn2 -- b/RConn1
  Three-Phase Series RLC Branch4/LConn1 -- a/RConn1

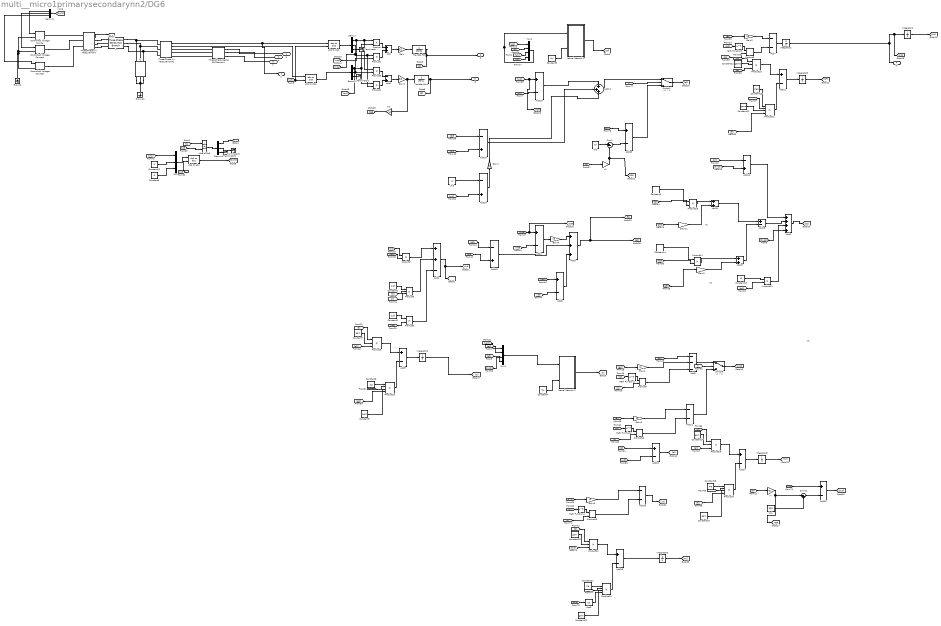
== system multi__micro1primarysecondarynn2/DG6 ==
  note: SE
  note: SE
  note: SE
  Abs3 : Abs
  Add : Sum
  Add{1,13,15..16,19} (5 alike) : Sum  Inputs=-+
  Add{4,6,9..10,12,18,22..26} (11 alike) : Sum  Inputs=+-
  Add11 : Sum  Inputs=+++
  Add14 : Sum
  Add17 : Sum
  Add2 : Sum  Inputs=++-
  Add20 : Sum  Inputs=--
  Add21 : Sum  Inputs=--
  Add3 : Sum  Inputs=+++
  Add5 : Sum  Inputs=++++
  Add7 : Sum  Inputs=--
  Add8 : Sum  Inputs=---
  C : powerlib/Elements/Three-Phase Series RLC Branch  LConnTagsString=A|B|C  RConnTagsString=A|B|C  BranchType=C  Resistance=1  Inductance=1e-3  Capacitance=cf  Measurements=None
  Constant1 : Constant  Value=1/cf
  Constant10 : Constant  Value=0
  Constant11 : Constant  Value=gamp
  Constant12 : Constant  Value=gamp
  Constant13 : Constant  Value=sigp
  Constant14 : Constant  Value=-31.446
  Constant15 : Constant  Value=k1
  Constant{7,9,17,19..20,22} (6 alike) : Constant  Value=gam
  Constant18 : Constant  Value=sig
  Constant2 : Constant  Value=1/cf
  Constant21 : Constant  Value=sig
  Constant3 : Constant  Value=Mu
  Constant4 : Constant  Value=Mu
  Constant5 : Constant  Value=-31.446
  Constant6 : Constant  Value=0
  Constant8 : Constant  Value=sig
  Controlled Voltage Source : powerlib/Electrical Sources/Controlled Voltage Source  Initialize=on  Source_Type=AC  Amplitude=0  Phase=0  Frequency=0  Measurements=None
  Controlled Voltage Source1 : powerlib/Electrical Sources/Controlled Voltage Source  Initialize=on  Source_Type=AC  Amplitude=0  Phase=0  Frequency=0  Measurements=None
  Controlled Voltage Source2 : powerlib/Electrical Sources/Controlled Voltage Source  Initialize=on  Source_Type=AC  Amplitude=0  Phase=0  Frequency=0  Measurements=None
  Demux{,1,3..4} (4 alike) : Demux  Outputs=3
  Gain : Gain  Gain=3/2
  Gain1 : Gain  Gain=3/2
  Gain11 : Gain  Gain=31.446
  Gain2 : Gain  Gain=k3
  Gain3 : Gain  Gain=31.446
  Gain4 : Gain  Gain=k2
  Gain5 : Gain  Gain=k5
  Gain7 : Gain  Gain=k5
  Gain8 : Gain  Gain=k2
  Gain9 : Gain  Gain=k2
  Ground : powerlib/Elements/Ground  LConnTagsString=a
  Ground1 : powerlib/Elements/Ground  LConnTagsString=a
  Integrator1 : Integrator  UpperSaturationLimit=321  LowerSaturationLimit=314.16
  Integrator{2..3,5..6} (4 alike) : Integrator  InitialCondition=zeros(16,1)  UpperSaturationLimit=314.16  ZeroCross=off
  Integrator4 : Integrator  UpperSaturationLimit=314.16  ZeroCross=off
  L : powerlib/Elements/Three-Phase Series RLC Branch  LConnTagsString=A|B|C  RConnTagsString=A|B|C  BranchType=RL  Resistance=0.1  Inductance=lf  Capacitance=1e-6  Measurements=None
  Math Function{1..4} (4 alike) : Math  Operator=transpose  OutputSignalType=real  SaturateOnIntegerOverflow=on
  Mux : Mux  Inputs=3
  Mux1 : Mux
  Mux2 : Mux
  Neural Network 1 : MATLAB Function  TreatAsAtomicUnit=on
  Neural Network 2 : MATLAB Function  TreatAsAtomicUnit=on
  Product{,1,3..4} (4 alike) : Product  RndMeth=Zero
  Product{10,12,17,20} (4 alike) : Product  Inputs=4
  Product{2,6,11,14..15} (5 alike) : Product
  Product{5,8,13,18,21} (5 alike) : Product  Inputs=3
  Product{7,9,16,19} (4 alike) : Product  Multiplication=Matrix(*)
  Sum1 : Sum  Inputs=|+-
  Sum11 : Sum  Inputs=|-+
  Switch1 : Switch  Criteria=u2 > Threshold
  Switch3 : Switch  Criteria=u2 > Threshold
  Terminator{,1..3} (4 alike) : Terminator
  Three-Phase Series RLC Branch4 : powerlib/Elements/Three-Phase Series RLC Branch  LConnTagsString=A|B|C  RConnTagsString=A|B|C  BranchType=RL  Resistance=rc  Inductance=Lc  Capacitance=1e-6  Measurements=None
  Three-Phase V-I Measurement : powerlib/Measurements/Three-Phase V-I Measurement  VoltageMeasurement=phase-to-ground  SetLabelV=off  LabelV=Vabc  Vpu=off  VpuLL=off  CurrentMeasurement=yes  SetLabelI=off  LabelI=Iabc  Ipu=off  Pbase=100e6  Vbase=500e3  OutputType=Complex  PhasorSimulation=off  PSBequivalent=0
  Three-Phase V-I Measurement1 : powerlib/Measurements/Three-Phase V-I Measurement  VoltageMeasurement=phase-to-ground  SetLabelV=off  LabelV=Vabc  Vpu=off  VpuLL=off  CurrentMeasurement=yes  SetLabelI=off  LabelI=Iabc  Ipu=off  Pbase=100e6  Vbase=500e3  OutputType=Complex  PhasorSimulation=off  PSBequivalent=0
  Transfer Fcn : TransferFcn  Denominator=[td 1]
  Transfer Fcn1 : TransferFcn  Denominator=[td 1]
  Un1 : Constant  Value=325
  Un2 : Constant  Value=wn
  Un3 : Constant  Value=wn
  abc to dq0 : powerlib_meascontrol/Transformations/abc to dq0  Alignment=90 degrees behind phase A axis
  abc to dq1 : powerlib_meascontrol/Transformations/abc to dq0  Alignment=90 degrees behind phase A axis
  abc to dq3 : powerlib_meascontrol/Transformations/abc to dq0  Alignment=90 degrees behind phase A axis
  dq0 to abc : powerlib_meascontrol/Transformations/dq0 to abc  Alignment=90 degrees behind phase A axis
  m : Gain  Gain=nq1
  m1 : Gain  Gain=nq1
  n1 : Gain  Gain=mp1
  a : PMIOPort  Tag=PMCPort  Port=1  Side=Right
  b : PMIOPort  Tag=PMCPort  Port=2  Side=Right
  c : PMIOPort  Tag=PMCPort  Port=3  Side=Right
  U : Outport
  P : Outport  Port=2
  Q : Outport  Port=3
  f1 : Outport  Port=4
  tag scope: E6=global, MP6=global, NQ6=global, Q66=global, dv6=global, vod6=global, w16=global
  wires:
  [PWM] -> Demux4/1
  Three-Phase V-I Measurement1/1 -> U/1, abc to dq1/1
  Demux/1 -> [vod], Product/1, Product3/1
  Demux1/1 -> [iod], Product/2, Product4/1
  Demux/2 -> [voq], Product1/1, Product4/2
  Demux1/2 -> Product1/2, Product3/2
  Product/1 -> Add/1
  Product1/1 -> Add/2
  Product3/1 -> Add1/1
  Product4/1 -> Add1/2
  [wt] -> abc to dq1/2, abc to dq0/2
  Demux4/1 -> Controlled Voltage Source/1
  Demux4/2 -> Controlled Voltage Source1/1
  Demux4/3 -> Controlled Voltage Source2/1
  Three-Phase V-I Measurement/2 -> [IL]
  Add/1 -> Gain/1
  Gain/1 -> Transfer Fcn/1
  Add1/1 -> Gain1/1
  Gain1/1 -> m1/1, Transfer Fcn1/1
  abc to dq1/1 -> Demux/1
  abc to dq0/1 -> Demux1/1
  Demux/3 -> Terminator/1
  Demux1/3 -> Terminator1/1
  [vod] -> [vod6], Add4/1
  Gain4/1 -> Add8/2
  [e2] -> Gain4/1
  [S] -> Product7/2
  [W] -> Math Function1/1
  Math Function1/1 -> Product7/1
  Product7/1 -> Add8/3
  [S] -> Product8/1
  Constant7/1 -> Product8/2
  [e2] -> Product8/3
  Product8/1 -> Add9/1
  Constant8/1 -> Product10/1
  [W] -> Product10/2
  Product10/1 -> Add9/2
  Constant9/1 -> Product10/3
  Add9/1 -> Integrator2/1
  [vod5] -> Add4/2
  [IL] -> abc to dq3/1
  Demux3/1 -> [Id]
  Demux3/2 -> Terminator3/1
  [wt] -> abc to dq3/2
  Mux/1 -> dq0 to abc/1
  [wt] -> dq0 to abc/2
  abc to dq3/1 -> Demux3/1
  dq0 to abc/1 -> [PWM]
  Demux3/3 -> Terminator2/1
  [vn1] -> Mux/1
  Constant10/1 -> Mux/2
  Constant6/1 -> Mux/3
  Transfer Fcn/1 -> P/1, [P]
  Transfer Fcn1/1 -> Q/1, [Q]
  [w1] -> Mux1/1
  [ef] -> Mux1/2
  [w1] -> Mux1/3
  [MP2] -> Mux1/4
  [w1] -> [w16], Add10/1
  [w13] -> Add10/2
  [Sf] -> Product13/1
  Constant12/1 -> Product13/2
  [ef] -> Product13/3
  Product13/1 -> Add12/1
  Constant13/1 -> Product12/1
  [Wf] -> Product12/2
  Product12/1 -> Add12/2
  Constant11/1 -> Product12/3
  Add12/1 -> Integrator3/1
  Integrator3/1 -> [Wf]
  Three-Phase V-I Measurement1/2 -> abc to dq0/1
  Add10/1 -> Add11/1
  [MP3] -> Add13/1
  [MP4] -> Add13/2
  Add13/1 -> Add11/2
  [NQ5] -> Add15/1
  [NQ6] -> Add15/2
  Add15/1 -> Add3/2
  [e1] -> Add8/1
  Add4/1 -> Gain5/1
  Gain5/1 -> Add3/1
  [vod] -> Mux2/1
  [e1] -> Mux2/2
  [dvodi] -> Mux2/3
  [e2] -> Mux2/4
  Constant5/1 -> Product15/1
  [NQ6] -> Product15/2
  Product15/1 -> Add14/1
  [Q66] -> Gain11/1
  Constant14/1 -> Product14/1
  [NQ5] -> Product14/2
  Product14/1 -> Add17/1
  [Q55] -> Gain3/1
  Add17/1 -> Add18/2
  Add14/1 -> Add18/1
  Gain3/1 -> Add17/2
  Gain11/1 -> Add14/2
  Add18/1 -> Add5/2
  Constant15/1 -> Product11/1
  [e1] -> Product11/2
  Product11/1 -> Add5/3
  [dv5] -> Add16/1
  Add16/1 -> Add5/1
  [dvodi] -> Add16/2
  [vod] -> Add6/1
  [vref] -> Add6/2
  Add6/1 -> Add3/3
  m1/1 -> [Q66]
  Un3/1 -> Add19/1
  [w1] -> Add19/2
  Add19/1 -> Gain7/1
  Gain7/1 -> Add11/3
  Neural Network 1/1(Sz1) -> [Sf]
  [e2] -> Product10/4
  [ef] -> Gain2/1
  [Sf] -> Product9/2
  [Wf] -> Math Function3/1
  Math Function3/1 -> Product9/1
  Gain2/1 -> Add7/1
  Product9/1 -> Add7/2
  Add7/1 -> Integrator1/1
  [ef] -> Product12/4
  Neural Network 2/1(Sz1) -> [S]
  Constant4/1 -> Neural Network 2/2(mu)
  Mux2/1 -> Neural Network 2/1(X)
  Constant3/1 -> Neural Network 1/2(mu)
  Mux1/1 -> Neural Network 1/1(X)
  Add3/1 -> [E6], [e1]
  Add5/1 -> [e2]
  Integrator4/1 -> [wt]
  [ti] -> Switch3/2
  Add8/1 -> Switch3/1
  Switch3/1 -> [vn1]
  [el] -> Gain8/1
  [S] -> Product16/2
  [Wl] -> Math Function2/1
  Math Function2/1 -> Product16/1
  Product16/1 -> Add21/2
  Gain8/1 -> Add21/1
  Add21/1 -> Switch3/3
  [Id] -> Add22/1
  [vd] -> Add22/2
  Add22/1 -> [el]
  [S] -> Product18/1
  Constant17/1 -> Product18/2
  [el] -> Product18/3
  Product18/1 -> Add24/1
  Constant18/1 -> Product17/1
  [Wl] -> Product17/2
  Product17/1 -> Add24/2
  Constant19/1 -> Product17/3
  Add24/1 -> Integrator5/1
  Integrator5/1 -> [Wl]
  [el] -> Product17/4
  [vod] -> Add25/1
  Add25/1 -> [evd]
  Sum11/1 -> Add25/2
  [Q] -> m/1
  Un1/1 -> Sum11/2
  m/1 -> [NQ6], Sum11/1
  [evd] -> Gain9/1
  [S] -> Product19/2
  [Wv] -> Math Function4/1
  Math Function4/1 -> Product19/1
  Product19/1 -> Add20/2
  Gain9/1 -> Add20/1
  Add20/1 -> [vd]
  [S] -> Product21/1
  Constant20/1 -> Product21/2
  [evd] -> Product21/3
  Product21/1 -> Add26/1
  Constant21/1 -> Product20/1
  [Wl] -> Product20/2
  Product20/1 -> Add26/2
  Constant22/1 -> Product20/3
  Abs3/1 -> Product20/4
  [evd] -> Abs3/1
  Add26/1 -> Integrator6/1
  Integrator6/1 -> [Wv]
  Integrator2/1 -> [W]
  [w1] -> Product2/1
  [voq] -> Product2/2
  Product2/1 -> Add2/1
  Constant1/1 -> Product5/1
  [Id] -> Product5/2
  Product5/1 -> Add2/2
  Constant2/1 -> Product6/1
  [iod] -> Product6/2
  Product6/1 -> Add2/3
  Add2/1 -> [dvodi], [dv6]
  [rr] -> Product5/3
  Integrator1/1 -> [w1], Integrator4/1, f1/1
  [P] -> n1/1
  Un2/1 -> Sum1/1  "f"
  n1/1 -> [MP6], Sum1/2
  Sum1/1 -> Add23/2
  [w1] -> Add23/1
  Add11/1 -> Switch1/1
  [ti] -> Switch1/2
  Switch1/1 -> [ef]
  Add23/1 -> Switch1/3
  [dvodi] -> Add5/4
  connections:
  C/RConn1 -- Ground1/LConn1 -- C/RConn3 -- C/RConn2
  L/RConn2 -- Three-Phase V-I Measurement1/LConn2 -- C/LConn2
  L/RConn1 -- Three-Phase V-I Measurement1/LConn1 -- C/LConn1
  L/RConn3 -- Three-Phase V-I Measurement1/LConn3 -- C/LConn3
  Controlled Voltage Source/LConn1 -- Controlled Voltage Source1/LConn1 -- Ground/LConn1 -- Controlled Voltage Source2/LConn1
  Three-Phase V-I Measurement/LConn1 -- Controlled Voltage Source/RConn1
  Controlled Voltage Source1/RConn1 -- Three-Phase V-I Measurement/LConn2
  Controlled Voltage Source2/RConn1 -- Three-Phase V-I Measurement/LConn3
  Three-Phase V-I Measurement/RConn1 -- L/LConn1
  Three-Phase V-I Measurement/RConn2 -- L/LConn2
  Three-Phase V-I Measurement/RConn3 -- L/LConn3
  Three-Phase Series RLC Branch4/RConn1 -- Three-Phase V-I Measurement1/RConn1
  Three-Phase Series RLC Branch4/RConn2 -- Three-Phase V-I Measurement1/RConn2
  Three-Phase Series RLC Branch4/RConn3 -- Three-Phase V-I Measurement1/RConn3
  Three-Phase Series RLC Branch4/LConn3 -- c/RConn1
  Three-Phase Series RLC Branch4/LConn2 -- b/RConn1
  Three-Phase Series RLC Branch4/LConn1 -- a/RConn1
